simulink model "Cascade_Motor_Controller"  (R2023b)
settings: Solver=VariableStepAuto  StartTime=0.0  StopTime=3  RelTol=1e-3
values from neighbouring files (symbols this model uses):
  B_eq_1 = J_eq_1 / t    (= 0.00468910616378)    [Cascade_Motor_Controller.m]
  current_ref = 25    [Cascade_Motor_Controller.m]
  degree_ref = 90    [Cascade_Motor_Controller.m]
  J_eq_1 = J_eq + 1/a*n^2*J_load    (= 1.76310391758e-05)    [Cascade_Motor_Controller.m]
  Ka_c = 1/Kp_c    (= 1.20999748321)    [Cascade_Motor_Controller.m]
  Ka_s = 1/Kp_s    (= 0.380774744139)    [Cascade_Motor_Controller.m]
  Kd_p = wcp/wcs    (= 0.1)    [Cascade_Motor_Controller.m]
  Ke = Kt    (= 0.0683)    [Cascade_Motor_Controller.m]
  Ki_c = Ra*wcc    (= 2210.56)    [Cascade_Motor_Controller.m]
  Ki_s = (1/n)*B_eq_1*wcs/Kt    (= 698.46398928)    [Cascade_Motor_Controller.m]
  Kp_c = La*wcc    (= 0.826448)    [Cascade_Motor_Controller.m]
  Kp_p = wcp    (= 12.56)    [Cascade_Motor_Controller.m]
  Kp_s = (1/n)*J_eq_1*wcs/Kt    (= 2.62622459969)    [Cascade_Motor_Controller.m]
  Kt = 68.3*10^-3    (= 0.0683)    [Cascade_Motor_Controller.m]
  La = 0.658*10^-3    (= 0.000658)    [Cascade_Motor_Controller.m]
  n = N1/N2    (= 0.0123456790123)    [Cascade_Motor_Controller.m]
  Ra = 1.76    [Cascade_Motor_Controller.m]
  speed_ref = 5    [Cascade_Motor_Controller.m]
  Tl = 0    [Cascade_Motor_Controller.m]
libraries: simulink_extras x2
settings Model: Creator=jhpark  LastModifiedBy=jhpark

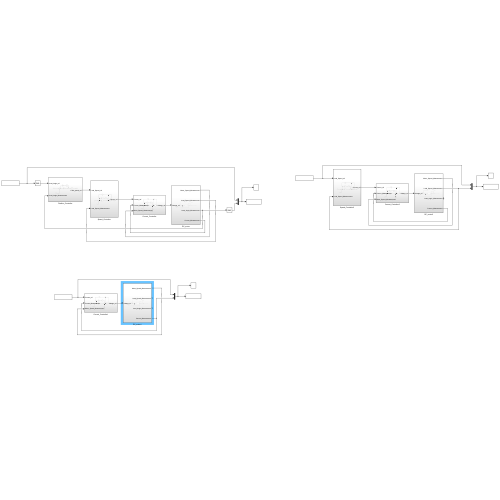
[thumbnail: Simulink's stored preview of the top-level diagram]
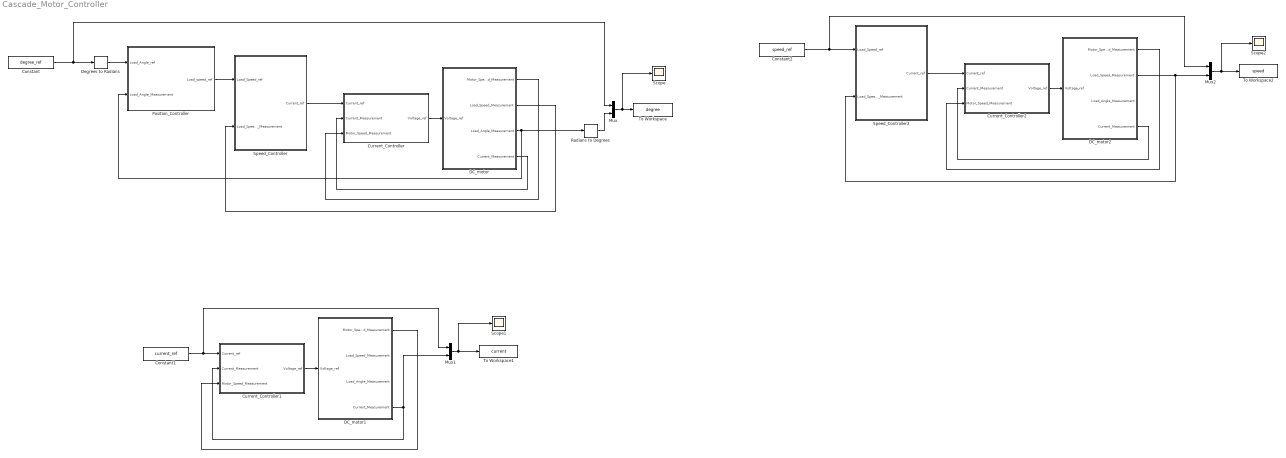
== system Cascade_Motor_Controller ==
  Constant : Constant  Value=degree_ref
  Constant1 : Constant  Value=current_ref
  Constant2 : Constant  Value=speed_ref
  Current_Controller : Subsystem
  Current_Controller1 : Subsystem
  Current_Controller2 : Subsystem
  DC_motor : Subsystem
  DC_motor1 : Subsystem
  DC_motor2 : Subsystem
  Degrees to Radians : simulink_extras/Transformations/Degrees to Radians
  Mux : Mux  Inputs=2
  Mux1 : Mux  Inputs=2
  Mux2 : Mux  Inputs=2
  Position_Controller : Subsystem
  Radians to Degrees : simulink_extras/Transformations/Radians to Degrees
  Scope : Scope
  Scope1 : Scope
  Scope2 : Scope
  Speed_Controller : Subsystem
  Speed_Controller2 : Subsystem
  To Workspace : ToWorkspace  VariableName=degree  SampleTime=-1
  To Workspace1 : ToWorkspace  VariableName=current  SampleTime=-1
  To Workspace2 : ToWorkspace  VariableName=speed  SampleTime=-1
  wires:
  Current_Controller/1(Voltage_ref) -> DC_motor/1(Voltage_ref)
  DC_motor/3(Load_Angle_Measurement) -> Radians to Degrees/1, Position_Controller/2(Load_Angle_Measurement)
  DC_motor/2(Load_Speed_Measurement) -> Speed_Controller/2(Load_Speed_Measurement)
  Mux/1 -> Scope/1, To Workspace/1
  DC_motor/1(Motor_Speed_Measurement) -> Current_Controller/3(Motor_Speed_Measurement)
  Speed_Controller/1(Current_ref) -> Current_Controller/1(Current_ref)
  Radians to Degrees/1 -> Mux/2
  DC_motor/4(Current_Measurement) -> Current_Controller/2(Current_Measurement)
  Position_Controller/1(Load_speed_ref) -> Speed_Controller/1(Load_Speed_ref)
  Degrees to Radians/1 -> Position_Controller/1(Load_Angle_ref)
  Constant/1 -> Mux/1, Degrees to Radians/1
  Mux1/1 -> To Workspace1/1, Scope1/1
  Constant1/1 -> Current_Controller1/1(Current_ref), Mux1/1
  Current_Controller1/1(Voltage_ref) -> DC_motor1/1(Voltage_ref)
  DC_motor1/4(Current_Measurement) -> Current_Controller1/2(Current_Measurement), Mux1/2
  DC_motor1/1(Motor_Speed_Measurement) -> Current_Controller1/3(Motor_Speed_Measurement)
  Mux2/1 -> To Workspace2/1, Scope2/1
  Constant2/1 -> Mux2/1, Speed_Controller2/1(Load_Speed_ref)
  Current_Controller2/1(Voltage_ref) -> DC_motor2/1(Voltage_ref)
  DC_motor2/4(Current_Measurement) -> Current_Controller2/2(Current_Measurement)
  DC_motor2/1(Motor_Speed_Measurement) -> Current_Controller2/3(Motor_Speed_Measurement)
  DC_motor2/2(Load_Speed_Measurement) -> Speed_Controller2/2(Load_Speed_Measurement), Mux2/2
  Speed_Controller2/1(Current_ref) -> Current_Controller2/1(Current_ref)

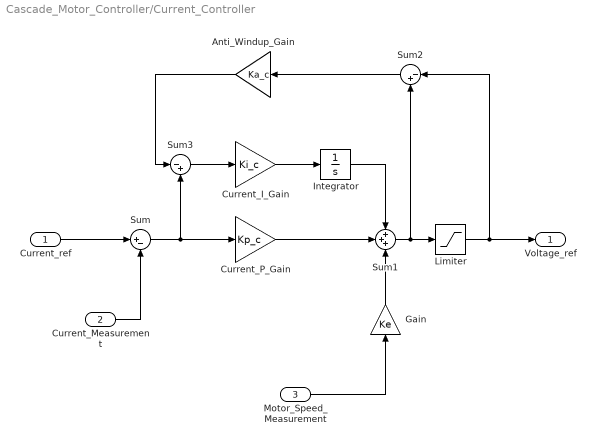
== system Cascade_Motor_Controller/Current_Controller ==
  Current_ref : Inport
  Current_Measurement : Inport  Port=2
  Motor_Speed_Measurement : Inport  Port=3
  Anti_Windup_Gain : Gain  Gain=Ka_c
  Current_I_Gain : Gain  Gain=Ki_c
  Current_P_Gain : Gain  Gain=Kp_c
  Gain : Gain  Gain=Ke
  Integrator : Integrator
  Limiter : Saturate  UpperLimit=48  LowerLimit=-48
  Sum : Sum  Inputs=|+-
  Sum1 : Sum  Inputs=+++
  Sum2 : Sum  Inputs=|-+
  Sum3 : Sum  Inputs=|-+
  Voltage_ref : Outport
  wires:
  Current_P_Gain/1 -> Sum1/2
  Sum/1 -> Sum3/2, Current_P_Gain/1
  Sum1/1 -> Sum2/2, Limiter/1
  Current_ref/1 -> Sum/1
  Current_Measurement/1 -> Sum/2
  Anti_Windup_Gain/1 -> Sum3/1
  Sum3/1 -> Current_I_Gain/1
  Gain/1 -> Sum1/3
  Integrator/1 -> Sum1/1
  Current_I_Gain/1 -> Integrator/1
  Sum2/1 -> Anti_Windup_Gain/1
  Limiter/1 -> Voltage_ref/1, Sum2/1
  Motor_Speed_Measurement/1 -> Gain/1

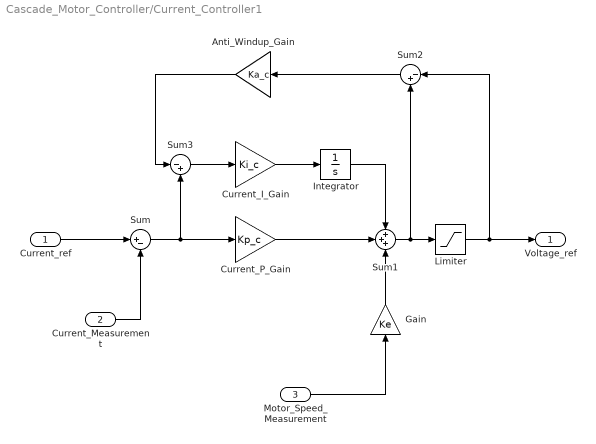
== system Cascade_Motor_Controller/Current_Controller1 ==
  Current_ref : Inport
  Current_Measurement : Inport  Port=2
  Motor_Speed_Measurement : Inport  Port=3
  Anti_Windup_Gain : Gain  Gain=Ka_c
  Current_I_Gain : Gain  Gain=Ki_c
  Current_P_Gain : Gain  Gain=Kp_c
  Gain : Gain  Gain=Ke
  Integrator : Integrator
  Limiter : Saturate  UpperLimit=48  LowerLimit=-48
  Sum : Sum  Inputs=|+-
  Sum1 : Sum  Inputs=+++
  Sum2 : Sum  Inputs=|-+
  Sum3 : Sum  Inputs=|-+
  Voltage_ref : Outport
  wires:
  Current_P_Gain/1 -> Sum1/2
  Sum/1 -> Sum3/2, Current_P_Gain/1
  Sum1/1 -> Sum2/2, Limiter/1
  Current_ref/1 -> Sum/1
  Current_Measurement/1 -> Sum/2
  Anti_Windup_Gain/1 -> Sum3/1
  Sum3/1 -> Current_I_Gain/1
  Gain/1 -> Sum1/3
  Integrator/1 -> Sum1/1
  Current_I_Gain/1 -> Integrator/1
  Sum2/1 -> Anti_Windup_Gain/1
  Limiter/1 -> Voltage_ref/1, Sum2/1
  Motor_Speed_Measurement/1 -> Gain/1

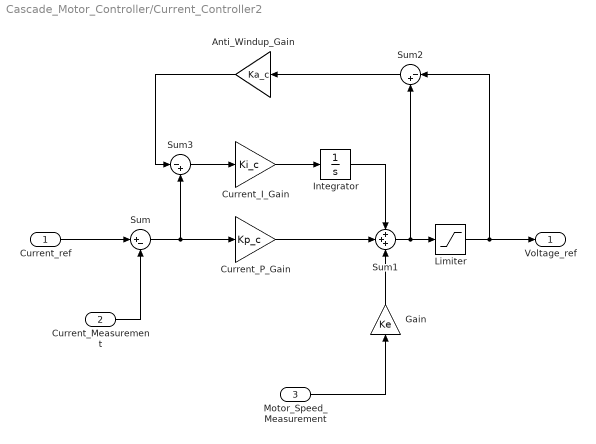
== system Cascade_Motor_Controller/Current_Controller2 ==
  Current_ref : Inport
  Current_Measurement : Inport  Port=2
  Motor_Speed_Measurement : Inport  Port=3
  Anti_Windup_Gain : Gain  Gain=Ka_c
  Current_I_Gain : Gain  Gain=Ki_c
  Current_P_Gain : Gain  Gain=Kp_c
  Gain : Gain  Gain=Ke
  Integrator : Integrator
  Limiter : Saturate  UpperLimit=48  LowerLimit=-48
  Sum : Sum  Inputs=|+-
  Sum1 : Sum  Inputs=+++
  Sum2 : Sum  Inputs=|-+
  Sum3 : Sum  Inputs=|-+
  Voltage_ref : Outport
  wires:
  Current_P_Gain/1 -> Sum1/2
  Sum/1 -> Sum3/2, Current_P_Gain/1
  Sum1/1 -> Sum2/2, Limiter/1
  Current_ref/1 -> Sum/1
  Current_Measurement/1 -> Sum/2
  Anti_Windup_Gain/1 -> Sum3/1
  Sum3/1 -> Current_I_Gain/1
  Gain/1 -> Sum1/3
  Integrator/1 -> Sum1/1
  Current_I_Gain/1 -> Integrator/1
  Sum2/1 -> Anti_Windup_Gain/1
  Limiter/1 -> Voltage_ref/1, Sum2/1
  Motor_Speed_Measurement/1 -> Gain/1

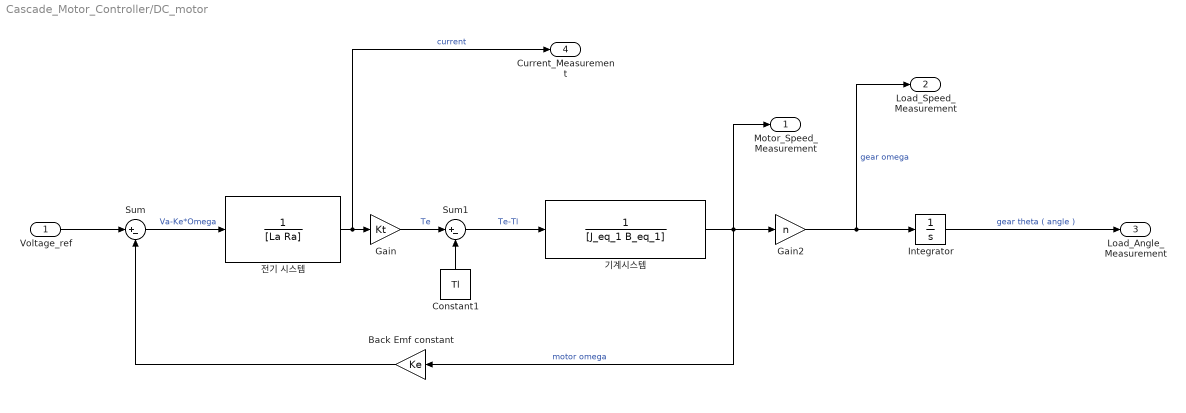
== system Cascade_Motor_Controller/DC_motor ==
  Voltage_ref : Inport
  Back Emf constant : Gain  Gain=Ke
  Constant1 : Constant  Value=Tl
  Gain : Gain  Gain=Kt
  Gain2 : Gain  Gain=n
  Integrator : Integrator
  Sum : Sum  Inputs=|+-
  Sum1 : Sum  Inputs=|+-
  기계시스템 : TransferFcn  Denominator=[J_eq_1 B_eq_1]
  전기 시스템 : TransferFcn  Denominator=[La Ra]
  Motor_Speed_Measurement : Outport
  Load_Speed_Measurement : Outport  Port=2
  Load_Angle_Measurement : Outport  Port=3
  Current_Measurement : Outport  Port=4
  wires:
  Back Emf constant/1 -> Sum/2
  기계시스템/1 -> Motor_Speed_Measurement/1, Gain2/1, Back Emf constant/1  "motor omega"
  Sum/1 -> 전기 시스템/1  "Va-Ke*Omega"
  전기 시스템/1 -> Current_Measurement/1, Gain/1  "current"
  Gain2/1 -> Load_Speed_Measurement/1, Integrator/1  "gear omega"
  Gain/1 -> Sum1/1  "Te"
  Integrator/1 -> Load_Angle_Measurement/1  "gear theta ( angle )"
  Constant1/1 -> Sum1/2
  Sum1/1 -> 기계시스템/1  "Te-Tl"
  Voltage_ref/1 -> Sum/1

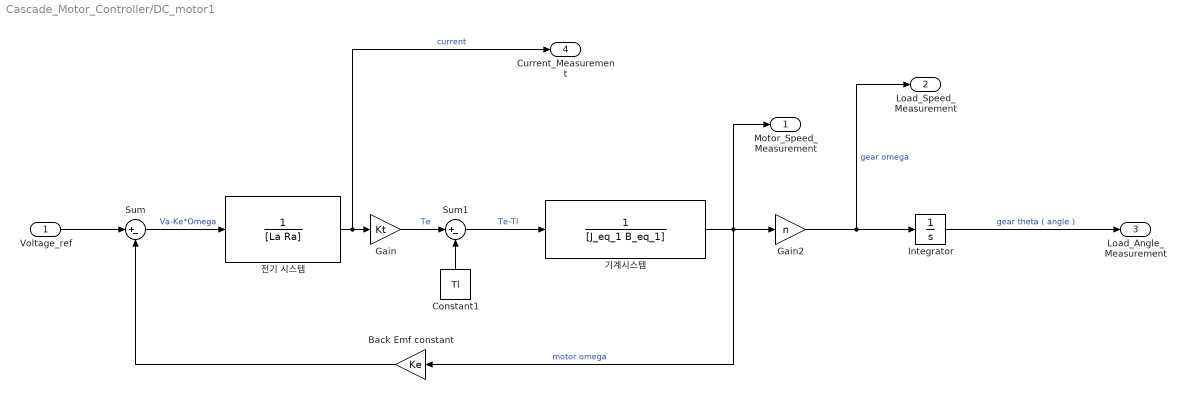
== system Cascade_Motor_Controller/DC_motor1 ==
  Voltage_ref : Inport
  Back Emf constant : Gain  Gain=Ke
  Constant1 : Constant  Value=Tl
  Gain : Gain  Gain=Kt
  Gain2 : Gain  Gain=n
  Integrator : Integrator
  Sum : Sum  Inputs=|+-
  Sum1 : Sum  Inputs=|+-
  기계시스템 : TransferFcn  Denominator=[J_eq_1 B_eq_1]
  전기 시스템 : TransferFcn  Denominator=[La Ra]
  Motor_Speed_Measurement : Outport
  Load_Speed_Measurement : Outport  Port=2
  Load_Angle_Measurement : Outport  Port=3
  Current_Measurement : Outport  Port=4
  wires:
  Back Emf constant/1 -> Sum/2
  기계시스템/1 -> Motor_Speed_Measurement/1, Gain2/1, Back Emf constant/1  "motor omega"
  Sum/1 -> 전기 시스템/1  "Va-Ke*Omega"
  전기 시스템/1 -> Current_Measurement/1, Gain/1  "current"
  Gain2/1 -> Load_Speed_Measurement/1, Integrator/1  "gear omega"
  Gain/1 -> Sum1/1  "Te"
  Integrator/1 -> Load_Angle_Measurement/1  "gear theta ( angle )"
  Constant1/1 -> Sum1/2
  Sum1/1 -> 기계시스템/1  "Te-Tl"
  Voltage_ref/1 -> Sum/1

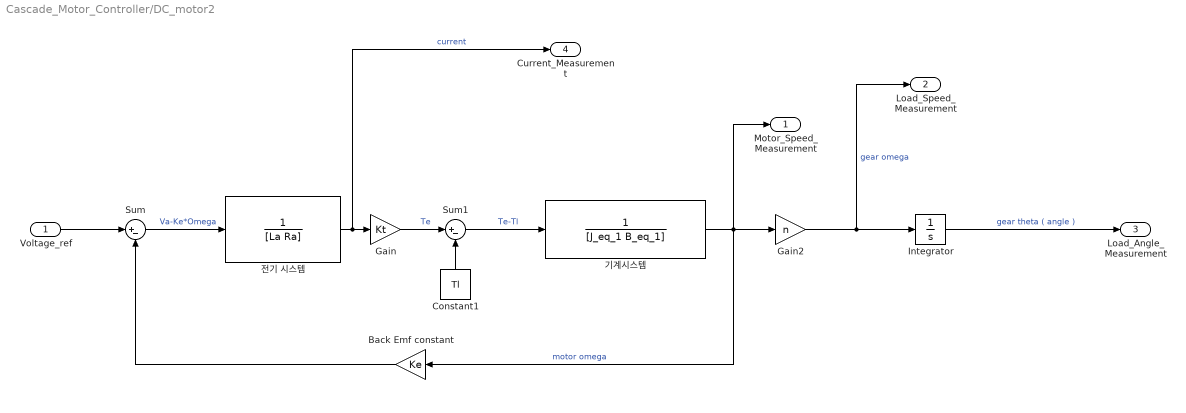
== system Cascade_Motor_Controller/DC_motor2 ==
  Voltage_ref : Inport
  Back Emf constant : Gain  Gain=Ke
  Constant1 : Constant  Value=Tl
  Gain : Gain  Gain=Kt
  Gain2 : Gain  Gain=n
  Integrator : Integrator
  Sum : Sum  Inputs=|+-
  Sum1 : Sum  Inputs=|+-
  기계시스템 : TransferFcn  Denominator=[J_eq_1 B_eq_1]
  전기 시스템 : TransferFcn  Denominator=[La Ra]
  Motor_Speed_Measurement : Outport
  Load_Speed_Measurement : Outport  Port=2
  Load_Angle_Measurement : Outport  Port=3
  Current_Measurement : Outport  Port=4
  wires:
  Back Emf constant/1 -> Sum/2
  기계시스템/1 -> Motor_Speed_Measurement/1, Gain2/1, Back Emf constant/1  "motor omega"
  Sum/1 -> 전기 시스템/1  "Va-Ke*Omega"
  전기 시스템/1 -> Current_Measurement/1, Gain/1  "current"
  Gain2/1 -> Load_Speed_Measurement/1, Integrator/1  "gear omega"
  Gain/1 -> Sum1/1  "Te"
  Integrator/1 -> Load_Angle_Measurement/1  "gear theta ( angle )"
  Constant1/1 -> Sum1/2
  Sum1/1 -> 기계시스템/1  "Te-Tl"
  Voltage_ref/1 -> Sum/1

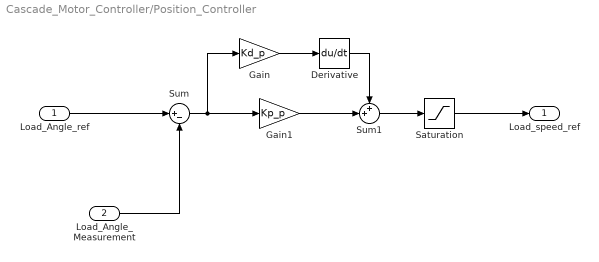
== system Cascade_Motor_Controller/Position_Controller ==
  Load_Angle_ref : Inport
  Load_Angle_Measurement : Inport  Port=2
  Derivative : Derivative
  Gain : Gain  Gain=Kd_p
  Gain1 : Gain  Gain=Kp_p
  Saturation : Saturate  UpperLimit=6140*pi/30  LowerLimit=-6140*pi/30  LinearizeAsGain=off
  Sum : Sum  Inputs=|+-
  Sum1 : Sum  Inputs=++|
  Load_speed_ref : Outport  VectorParamsAs1DForOutWhenUnconnected=off
  wires:
  Gain/1 -> Derivative/1
  Sum/1 -> Gain/1, Gain1/1
  Saturation/1 -> Load_speed_ref/1
  Derivative/1 -> Sum1/1
  Load_Angle_ref/1 -> Sum/1
  Gain1/1 -> Sum1/2
  Sum1/1 -> Saturation/1
  Load_Angle_Measurement/1 -> Sum/2

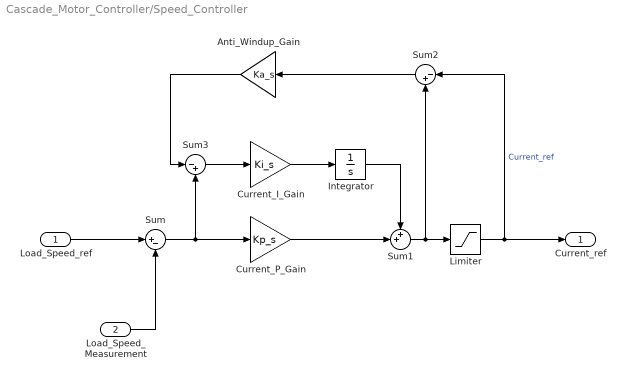
== system Cascade_Motor_Controller/Speed_Controller ==
  Load_Speed_ref : Inport
  Load_Speed_Measurement : Inport  Port=2
  Anti_Windup_Gain : Gain  Gain=Ka_s
  Current_I_Gain : Gain  Gain=Ki_s
  Current_P_Gain : Gain  Gain=Kp_s
  Integrator : Integrator
  Limiter : Saturate  UpperLimit=27.3  LowerLimit=-27.3
  Sum : Sum  Inputs=|+-
  Sum1 : Sum  Inputs=++|
  Sum2 : Sum  Inputs=|-+
  Sum3 : Sum  Inputs=|-+
  Current_ref : Outport
  wires:
  Sum3/1 -> Current_I_Gain/1
  Limiter/1 -> Current_ref/1, Sum2/1  "Current_ref"
  Sum1/1 -> Sum2/2, Limiter/1
  Sum2/1 -> Anti_Windup_Gain/1
  Sum/1 -> Sum3/2, Current_P_Gain/1
  Load_Speed_Measurement/1 -> Sum/2
  Anti_Windup_Gain/1 -> Sum3/1
  Current_I_Gain/1 -> Integrator/1
  Load_Speed_ref/1 -> Sum/1
  Integrator/1 -> Sum1/1
  Current_P_Gain/1 -> Sum1/2

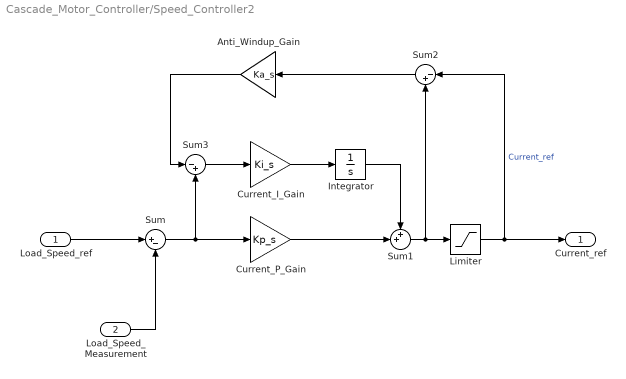
== system Cascade_Motor_Controller/Speed_Controller2 ==
  Load_Speed_ref : Inport
  Load_Speed_Measurement : Inport  Port=2
  Anti_Windup_Gain : Gain  Gain=Ka_s
  Current_I_Gain : Gain  Gain=Ki_s
  Current_P_Gain : Gain  Gain=Kp_s
  Integrator : Integrator
  Limiter : Saturate  UpperLimit=27.3  LowerLimit=-27.3
  Sum : Sum  Inputs=|+-
  Sum1 : Sum  Inputs=++|
  Sum2 : Sum  Inputs=|-+
  Sum3 : Sum  Inputs=|-+
  Current_ref : Outport
  wires:
  Sum3/1 -> Current_I_Gain/1
  Limiter/1 -> Current_ref/1, Sum2/1  "Current_ref"
  Sum1/1 -> Sum2/2, Limiter/1
  Sum2/1 -> Anti_Windup_Gain/1
  Sum/1 -> Sum3/2, Current_P_Gain/1
  Load_Speed_Measurement/1 -> Sum/2
  Anti_Windup_Gain/1 -> Sum3/1
  Current_I_Gain/1 -> Integrator/1
  Load_Speed_ref/1 -> Sum/1
  Integrator/1 -> Sum1/1
  Current_P_Gain/1 -> Sum1/2
